simulink model "voltage_droop_ideal_rectifier"  (R2020b)
settings: Solver=VariableStepAuto  StartTime=0.0  StopTime=1  RelTol=1e-3
undefined symbols (not defined in the file): DiscIntNeverNeededParam, droop1, droop2
libraries: fl_lib x13, nesl_utility x9, ee_lib x6, simulink x1
settings Model: Creator=gdudgeon  LastModifiedBy=gdudgeon

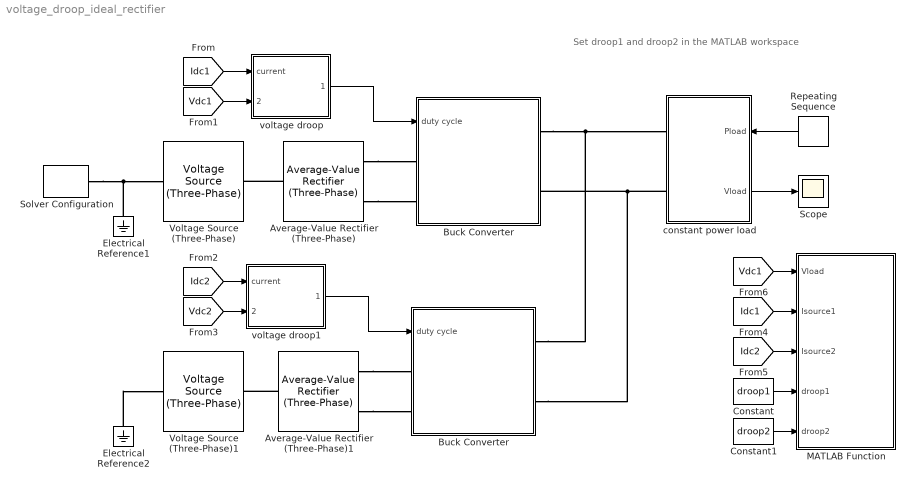
== system voltage_droop_ideal_rectifier ==
  note: Set droop1 and droop2 in the MATLAB workspace
  Average-Value Rectifier (Three-Phase) : ee_lib/Semiconductors & Converters/Converters/Average-Value Rectifier (Three-Phase)  VRated=4160 V  Pfixed=1e3 W
      settings: SourceProductBaseCode=PS  InternalSimscapePortConfiguration="{\"Bottom\":[],\"Left\":[{\"id\":\"N\",\"label\":\"~\",\"type\":\"foundation.electrical.three_phase\"}],\"Right\":[{\"id\":\"p\",\"label\":\"+\",\"type\":\"foundation.electrical.electrical\"},{\"id\":\"n\",\"label\":\"-\",\"type\":\"foundation.electrical.electrical\"}],\"Top\":[]}"
  Average-Value Rectifier (Three-Phase)1 : ee_lib/Semiconductors & Converters/Converters/Average-Value Rectifier (Three-Phase)  VRated=4160 V  Pfixed=1e3 W
      settings: SourceProductBaseCode=PS  InternalSimscapePortConfiguration="{\"Bottom\":[],\"Left\":[{\"id\":\"N\",\"label\":\"~\",\"type\":\"foundation.electrical.three_phase\"}],\"Right\":[{\"id\":\"p\",\"label\":\"+\",\"type\":\"foundation.electrical.electrical\"},{\"id\":\"n\",\"label\":\"-\",\"type\":\"foundation.electrical.electrical\"}],\"Top\":[]}"
  Buck Converter : Subsystem
  "Buck Converter " : Subsystem
  Constant : Constant  Value=droop1
  Constant1 : Constant  Value=droop2
  Electrical Reference1 : fl_lib/Electrical/Electrical Elements/Electrical Reference
  Electrical Reference2 : fl_lib/Electrical/Electrical Elements/Electrical Reference
  MATLAB Function : MATLAB Function  TreatAsAtomicUnit=on  SystemSampleTime=Tanim  mask(Machine Rotor Animation){Tanim=0.01}
      mask prompts: Tanim "Animation Rate [s]"
      mask help: This block animates permanent magnet inside a stator. The "thetaRotor" input is the angle of the rotor. The "phase" parameter must be defined in the workspace and selects the energized coil in the stator.
  Repeating Sequence : simulink/Sources/Repeating Sequence  rep_seq_t=[0 1 2]  rep_seq_y=[1e-3 1 1]
  Scope : Scope
  Solver Configuration : nesl_utility/Solver Configuration  PhysicalDomain=network_engine_domain  SubClassName=solver  LeftPortType=input  RightPortType=generic  Tones=[]  Harmonics=[]  SimulateNoise=off  Profile=off  UseLocalSampling=off  EnableSwitchedLinearOptims=on  FrequencyDomain=off  UseCCode=off  RelTol=0.001  AbsTol=1e-06  MinStep=1e-09  ToWorkspace=off  RevertToSquareIcSolve=off  NumHomotopyIterations=100  PhasorMode=off  PhasorModeNumHarmonics=1  DoDC=off  ResidualTolerance=1e-09  UseLocalSolver=on  LocalSolverChoice=NE_BACKWARD_EULER_ADVANCER  LocalSolverSampleTime=5e-5  DoFixedCost=on  MaxNonlinIter=3  MaxModeIter=2  ComputeImpulses=off  ImpulseIterations=2  LinearAlgebra=auto  EquationFormulation=NE_TIME_EF  DelaysMemoryBudget=1024  AutomaticFiltering=on  FilteringTimeConstant=0.001  PartitionStorageMethod=AS_NEEDED  PartitionMemoryBudget=1024  PartitionMethod=ROBUST
  Voltage Source (Three-Phase) : ee_lib/Sources/Voltage Source (Three-Phase)  vline_rms=1 V  shift=0 deg  freq=60 Hz  impedance_option=2  SShortCircuit=1e6 V*A  XR=15  R=1e-5 Ohm  L=3.97e-4 H  G_parasitic=0 1/Ohm  harmonic_option=0  harmonic_orders=[5, 7, 11, 13]  harmonic_ratios=[.1, .1, .1, .1]  I_specify=off  I_priority=None  I=[ 0 0 0 ] A  I_nominal_specify=off  I_nominal_unit=A  I_nominal_value=1
      settings: SourceProductBaseCode=PS
  Voltage Source (Three-Phase)1 : ee_lib/Sources/Voltage Source (Three-Phase)  vline_rms=1 V  shift=0 deg  freq=60 Hz  impedance_option=2  SShortCircuit=1e6 V*A  XR=15  R=1e-5 Ohm  L=3.97e-4 H  G_parasitic=0 1/Ohm  harmonic_option=0  harmonic_orders=[5, 7, 11, 13]  harmonic_ratios=[.1, .1, .1, .1]  I_specify=off  I_priority=None  I=[ 0 0 0 ] A  I_nominal_specify=off  I_nominal_unit=A  I_nominal_value=1
      settings: SourceProductBaseCode=PS
  constant power load : Subsystem
      settings: PortSchema="{\"entries\":[{\"content\":{\"sides\":[{\"content\":{\"connectorIds\":[\"LConn1\",\"LConn2\"]},\"type\":\"ConnectorPlacement.EquallySpacedRectSide\",\"uuid\":\"ede3b789-4807-48db-8c98-272deebb1f90\"},{\"content\":{\"connectorIds\":[\"In1\",\"Out1\"],\"side\":\"RIGHT\"},\"type\":\"ConnectorPlacement.EquallySpacedRectSide\",\"uuid\":\"cedec5e8-adcb-43e2-ab37-681d5d79ce2a\"},{\"content\":{\"connectorIds\":[],\"side\":\"TOP\"},\"type\":\"ConnectorPlacement.EquallySpacedRectSide\",\"uuid\":\"08b52c53-b13a-4cd2-b8db-308d9ebd4277\"},{\"content\":{\"connectorIds\":[],\"side\":\"HIDDEN\"},\"type\":\"ConnectorPlacement.EquallySpacedRectSide\",\"uuid\":\"3f956204-c540-4879-b053-0f78777aeccb\"}]},\"type\":\"ConnectorPlacement.EquallySpacedConnector\",\"uuid\":\"42303a72-b7ff-4a69-b636-ebca1dcca68c\"}],\"packageUris\":[\"http://schema.mathworks.com/mf0/Connector/R2020b\"],\"version\":\"1.0\"}"
  voltage droop : Subsystem  mask{droop=droop1}
  voltage droop1 : Subsystem  mask{droop=droop2}
  wires:
  constant power load/1(Vload) -> Scope/1
  Repeating Sequence/1 -> constant power load/1(Pload)
  Constant/1 -> MATLAB Function/4(droop1)
  Constant1/1 -> MATLAB Function/5(droop2)
  [Idc1] -> voltage droop/1(current)
  [Vdc1] -> voltage droop/2(voltage)
  [Vdc2] -> voltage droop1/2(voltage)
  [Idc2] -> voltage droop1/1(current)
  [Idc2] -> MATLAB Function/3(Isource2)
  [Idc1] -> MATLAB Function/2(Isource1)
  [Vdc1] -> MATLAB Function/1(Vload)
  voltage droop/1(duty cycle) -> Buck Converter/1(duty cycle)
  voltage droop1/1(duty cycle) -> "Buck Converter "/1(duty cycle)
  connections:
  constant power load/LConn2 -- "Buck Converter "/RConn2 -- Buck Converter/RConn2
  Electrical Reference1/LConn1 -- Solver Configuration/RConn1 -- Voltage Source (Three-Phase)/LConn1
  Electrical Reference2/LConn1 -- Voltage Source (Three-Phase)1/LConn1
  Average-Value Rectifier (Three-Phase)/LConn1 -- Voltage Source (Three-Phase)/RConn1
  Average-Value Rectifier (Three-Phase)1/LConn1 -- Voltage Source (Three-Phase)1/RConn1
  Average-Value Rectifier (Three-Phase)1/RConn1 -- "Buck Converter "/LConn1
  Average-Value Rectifier (Three-Phase)1/RConn2 -- "Buck Converter "/LConn2
  Buck Converter/RConn1 -- "Buck Converter "/RConn1 -- constant power load/LConn1
  Average-Value Rectifier (Three-Phase)/RConn1 -- Buck Converter/LConn1
  Average-Value Rectifier (Three-Phase)/RConn2 -- Buck Converter/LConn2

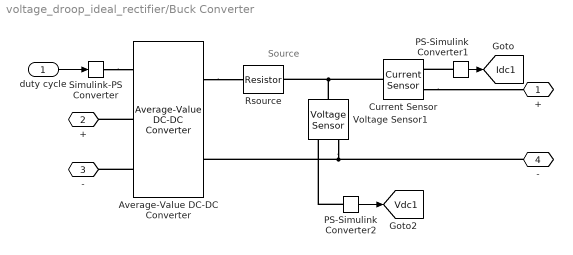
== system voltage_droop_ideal_rectifier/Buck Converter ==
  note: Source
  duty cycle : Inport
  Average-Value DC-DC Converter : ee_lib/Semiconductors & Converters/Converters/Average-Value DC-DC Converter  control_option=ee.enum.converters.controlinput.dutycycle  converter_type=ee.enum.converters.dcdctype.buck  efficiency_option=ee.enum.converters.efficiency.constant  efficiency_fixed=100  i_vec=[0, 2, 5] A  efficiency_vec=[90, 95, 98]
      settings: SourceProductBaseCode=PS  InternalSimscapePortConfiguration="{\"Bottom\":[],\"Left\":[{\"id\":\"DutyCycle\",\"label\":\"DutyCycle\",\"type\":\"input\"},{\"id\":\"p1\",\"label\":\"1+\",\"type\":\"foundation.electrical.electrical\"},{\"id\":\"n1\",\"label\":\"1-\",\"type\":\"foundation.electrical.electrical\"}],\"Right\":[{\"id\":\"p2\",\"label\":\"2+\",\"type\":\"foundation.electrical.electrical\"},{\"id\":\"n2\",\"label\":\"2-\",\"type\":\"foundation.electrical.electrical\"}],\"Top\":[]}"
  Current Sensor : fl_lib/Electrical/Electrical Sensors/Current Sensor
  PS-Simulink Converter1 : nesl_utility/PS-Simulink Converter  PhysicalDomain=network_engine_domain  SubClassName=ps_output  LeftPortType=input  RightPortType=output  PseudoPeriodic=off  Frequencies=[]  Unit=inherit  AffineConversion=off
  PS-Simulink Converter2 : nesl_utility/PS-Simulink Converter  PhysicalDomain=network_engine_domain  SubClassName=ps_output  LeftPortType=input  RightPortType=output  PseudoPeriodic=off  Frequencies=[]  Unit=inherit  AffineConversion=off
  Rsource : fl_lib/Electrical/Electrical Elements/Resistor  R=1e-2 Ohm  i_specify=off  i_priority=None  i=0 A  i_nominal_specify=off  i_nominal_unit=A  i_nominal_value=1  v_specify=off  v_priority=None  v=0 V  v_nominal_specify=off  v_nominal_unit=V  v_nominal_value=1
  Simulink-PS Converter : nesl_utility/Simulink-PS Converter  PhysicalDomain=network_engine_domain  SubClassName=ps_input  LeftPortType=input  RightPortType=output  PseudoPeriodic=off  Frequencies=[]  NoiseDistribution=none  NoiseParameters=[]  Unit=1  AffineConversion=off  FilteringAndDerivatives=provide  SimscapeFilterOrder=1  InputFilterTimeConstant=0.001  UdotUserProvided=0
  Voltage Sensor1 : fl_lib/Electrical/Electrical Sensors/Voltage Sensor
  "+ " : PMIOPort  Side=Right
  + : PMIOPort  Port=2  Side=Left
  - : PMIOPort  Port=3  Side=Left
  "- " : PMIOPort  Port=4  Side=Right
  tag scope: Idc1=global, Vdc1=global
  wires:
  PS-Simulink Converter2/1 -> [Vdc1]
  PS-Simulink Converter1/1 -> [Idc1]
  duty cycle/1 -> Simulink-PS Converter/1
  connections:
  Current Sensor/RConn2 -- "+ "/RConn1
  PS-Simulink Converter1/LConn1 -- Current Sensor/RConn1
  Voltage Sensor1/RConn2 -- "- "/RConn1 -- Average-Value DC-DC Converter/RConn2
  Average-Value DC-DC Converter/RConn1 -- Rsource/LConn1
  Current Sensor/LConn1 -- Voltage Sensor1/LConn1 -- Rsource/RConn1
  PS-Simulink Converter2/LConn1 -- Voltage Sensor1/RConn1
  Simulink-PS Converter/RConn1 -- Average-Value DC-DC Converter/LConn1
  Average-Value DC-DC Converter/LConn3 -- -/RConn1
  Average-Value DC-DC Converter/LConn2 -- +/RConn1

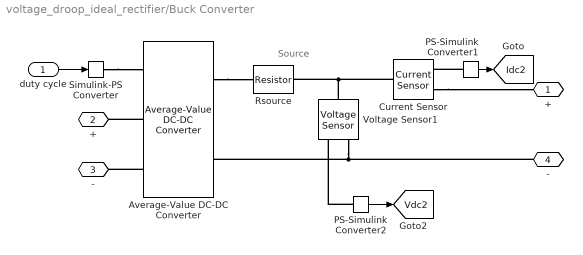
== system voltage_droop_ideal_rectifier/Buck Converter  ==
  note: Source
  duty cycle : Inport
  Average-Value DC-DC Converter : ee_lib/Semiconductors & Converters/Converters/Average-Value DC-DC Converter  control_option=ee.enum.converters.controlinput.dutycycle  converter_type=ee.enum.converters.dcdctype.buck  efficiency_option=ee.enum.converters.efficiency.constant  efficiency_fixed=100  i_vec=[0, 2, 5] A  efficiency_vec=[90, 95, 98]
      settings: SourceProductBaseCode=PS  InternalSimscapePortConfiguration="{\"Bottom\":[],\"Left\":[{\"id\":\"DutyCycle\",\"label\":\"DutyCycle\",\"type\":\"input\"},{\"id\":\"p1\",\"label\":\"1+\",\"type\":\"foundation.electrical.electrical\"},{\"id\":\"n1\",\"label\":\"1-\",\"type\":\"foundation.electrical.electrical\"}],\"Right\":[{\"id\":\"p2\",\"label\":\"2+\",\"type\":\"foundation.electrical.electrical\"},{\"id\":\"n2\",\"label\":\"2-\",\"type\":\"foundation.electrical.electrical\"}],\"Top\":[]}"
  Current Sensor : fl_lib/Electrical/Electrical Sensors/Current Sensor
  PS-Simulink Converter1 : nesl_utility/PS-Simulink Converter  PhysicalDomain=network_engine_domain  SubClassName=ps_output  LeftPortType=input  RightPortType=output  PseudoPeriodic=off  Frequencies=[]  Unit=inherit  AffineConversion=off
  PS-Simulink Converter2 : nesl_utility/PS-Simulink Converter  PhysicalDomain=network_engine_domain  SubClassName=ps_output  LeftPortType=input  RightPortType=output  PseudoPeriodic=off  Frequencies=[]  Unit=inherit  AffineConversion=off
  Rsource : fl_lib/Electrical/Electrical Elements/Resistor  R=1e-2 Ohm  i_specify=off  i_priority=None  i=0 A  i_nominal_specify=off  i_nominal_unit=A  i_nominal_value=1  v_specify=off  v_priority=None  v=0 V  v_nominal_specify=off  v_nominal_unit=V  v_nominal_value=1
  Simulink-PS Converter : nesl_utility/Simulink-PS Converter  PhysicalDomain=network_engine_domain  SubClassName=ps_input  LeftPortType=input  RightPortType=output  PseudoPeriodic=off  Frequencies=[]  NoiseDistribution=none  NoiseParameters=[]  Unit=1  AffineConversion=off  FilteringAndDerivatives=provide  SimscapeFilterOrder=1  InputFilterTimeConstant=0.001  UdotUserProvided=0
  Voltage Sensor1 : fl_lib/Electrical/Electrical Sensors/Voltage Sensor
  "+ " : PMIOPort  Side=Right
  + : PMIOPort  Port=2  Side=Left
  - : PMIOPort  Port=3  Side=Left
  "- " : PMIOPort  Port=4  Side=Right
  tag scope: Idc2=global, Vdc2=global
  wires:
  PS-Simulink Converter1/1 -> [Idc2]
  PS-Simulink Converter2/1 -> [Vdc2]
  duty cycle/1 -> Simulink-PS Converter/1
  connections:
  Average-Value DC-DC Converter/LConn2 -- +/RConn1
  Average-Value DC-DC Converter/LConn3 -- -/RConn1
  Simulink-PS Converter/RConn1 -- Average-Value DC-DC Converter/LConn1
  PS-Simulink Converter2/LConn1 -- Voltage Sensor1/RConn1
  Voltage Sensor1/LConn1 -- Rsource/RConn1 -- Current Sensor/LConn1
  Average-Value DC-DC Converter/RConn1 -- Rsource/LConn1
  "- "/RConn1 -- Average-Value DC-DC Converter/RConn2 -- Voltage Sensor1/RConn2
  PS-Simulink Converter1/LConn1 -- Current Sensor/RConn1
  Current Sensor/RConn2 -- "+ "/RConn1

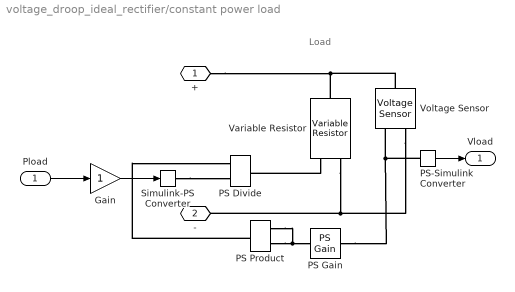
== system voltage_droop_ideal_rectifier/constant power load ==
  note: Load
  Pload : Inport
  Gain : Gain
  PS Divide : fl_lib/Physical Signals/Functions/PS Divide
      settings: SourceProductBaseCode=SS
  PS Gain : fl_lib/Physical Signals/Functions/PS Gain  gain=-1
  PS Product : fl_lib/Physical Signals/Functions/PS Product
  PS-Simulink Converter : nesl_utility/PS-Simulink Converter  PhysicalDomain=network_engine_domain  SubClassName=ps_output  LeftPortType=input  RightPortType=output  PseudoPeriodic=off  Frequencies=[]  Unit=inherit  AffineConversion=off
  Simulink-PS Converter : nesl_utility/Simulink-PS Converter  PhysicalDomain=network_engine_domain  SubClassName=ps_input  LeftPortType=input  RightPortType=output  PseudoPeriodic=off  Frequencies=[]  NoiseDistribution=none  NoiseParameters=[]  Unit=W  AffineConversion=off  FilteringAndDerivatives=provide  SimscapeFilterOrder=1  InputFilterTimeConstant=0.001  UdotUserProvided=0
  Variable Resistor : fl_lib/Electrical/Electrical Elements/Variable Resistor  Rmin=1 Ohm  i_specify=off  i_priority=None  i=0 A  i_nominal_specify=off  i_nominal_unit=A  i_nominal_value=1  v_specify=off  v_priority=None  v=0 V  v_nominal_specify=off  v_nominal_unit=V  v_nominal_value=1
  Voltage Sensor : fl_lib/Electrical/Electrical Sensors/Voltage Sensor
  + : PMIOPort  Side=Left
  - : PMIOPort  Port=2  Side=Left
  Vload : Outport
  wires:
  PS-Simulink Converter/1 -> Vload/1
  Pload/1 -> Gain/1
  Gain/1 -> Simulink-PS Converter/1
  connections:
  PS-Simulink Converter/LConn1 -- PS Gain/LConn1 -- Voltage Sensor/RConn1
  Variable Resistor/LConn1 -- PS Divide/RConn1
  Voltage Sensor/RConn2 -- -/RConn1 -- Variable Resistor/LConn2
  Voltage Sensor/LConn1 -- +/RConn1 -- Variable Resistor/RConn1
  Simulink-PS Converter/RConn1 -- PS Divide/LConn2
  PS Product/LConn1 -- PS Product/LConn2 -- PS Gain/RConn1
  PS Product/RConn1 -- PS Divide/LConn1

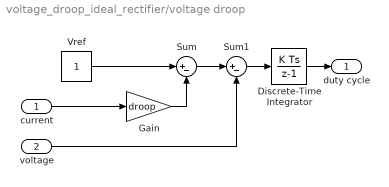
== system voltage_droop_ideal_rectifier/voltage droop ==
  current : Inport
  voltage : Inport  Port=2
  Discrete-Time Integrator : DiscreteIntegrator  gainval=1000  InitialCondition=0.5  SampleTime=-1  ICPrevOutput=DiscIntNeverNeededParam  ICPrevScaledInput=DiscIntNeverNeededParam
  Gain : Gain  Gain=droop
  Sum : Sum  Inputs=|+-
  Sum1 : Sum  Inputs=|+-
  Vref : Constant
  duty cycle : Outport
  wires:
  voltage/1 -> Sum1/2
  Sum1/1 -> Discrete-Time Integrator/1
  Vref/1 -> Sum/1
  Gain/1 -> Sum/2
  Sum/1 -> Sum1/1
  current/1 -> Gain/1
  Discrete-Time Integrator/1 -> duty cycle/1

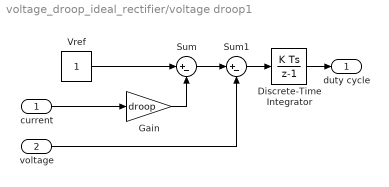
== system voltage_droop_ideal_rectifier/voltage droop1 ==
  current : Inport
  voltage : Inport  Port=2
  Discrete-Time Integrator : DiscreteIntegrator  gainval=1000  InitialCondition=0.5  SampleTime=-1  ICPrevOutput=DiscIntNeverNeededParam  ICPrevScaledInput=DiscIntNeverNeededParam
  Gain : Gain  Gain=droop
  Sum : Sum  Inputs=|+-
  Sum1 : Sum  Inputs=|+-
  Vref : Constant
  duty cycle : Outport
  wires:
  current/1 -> Gain/1
  Sum/1 -> Sum1/1
  Gain/1 -> Sum/2
  Vref/1 -> Sum/1
  Discrete-Time Integrator/1 -> duty cycle/1
  Sum1/1 -> Discrete-Time Integrator/1
  voltage/1 -> Sum1/2

== matlab function voltage_droop_ideal_rectifier/MATLAB Function ==
  data: Vload input; Isource1 input; Isource2 input; droop1 input; droop2 input
function plotDroop2(Vload,Isource1,Isource2,droop1,droop2)

persistent hf hp hp2 hp3


if isempty(hf)
    
    figure(1); clf(1); hold on;
    
    [hf,hp,hp2,hp3] = plotBackground(Vload,Isource1,Isource2,droop1,droop2);
  
    drawnow
    
else
    
    updateAnimation(hp,hp2,hp3,Vload,Isource1,Isource2);

    drawnow

end

end


function [hf,hp,hp2,hp3] = plotBackground(Vload,Isource1,Isource2,droop1,droop2)

hf = figure(1);hold on,grid %#ok<*DUALC>

hp = plot([0 1],[1 1]*Vload);xlabel('Power (pu)'),ylabel('Voltage (pu)')
hp2 = plot([1 1]*Isource1*Vload,[0.94 Vload],'k--');

hp3 = plot([1 1]*Isource2*Vload,[0.94 Vload],'k--');

plot([0 1],[1 1-droop1],'r');
plot([0 1],[1 1-droop2],'g');

coder.extrinsic('num2str')

title(['Droop1 = ',num2str(droop1),' : Droop2 = ',num2str(droop2)])


end

function  updateAnimation(hp,hp2,hp3,Vload,Isource1,Isource2)


set(hp,'YData',[1 1]*Vload);

set(hp2,'XData',[1 1]*Isource1*Vload);
set(hp2,'YData',[0.94 Vload]);

set(hp3,'XData',[1 1]*Isource2*Vload);
set(hp3,'YData',[0.94 Vload]);


end
